simulink model "Configuration3Code"  (R2021a)
settings: Solver=ode23t  StartTime=0.0  StopTime=60.1  FixedStep=0.05  RelTol=1e-3  EnableMultiTasking=on
model workspace (MAT data in the model file):
  mapForSim : object (value not decoded)
  occGrid : robotics.BinaryOccupancyGrid (value not decoded)
undefined symbols (not defined in the file): cellPose, FloorSurface, isoPoses, objectLevel, objectTypeArray, platformPoses, PlowSurface, Ref, RobotSurface, WallSurface, X, Y, Z
libraries: sm_lib x308, nesl_utility x151, simulink x70, RP_Simulator_Components x4
(part 15 of 15)

== matlab function Configuration3Code/BEST Robotics 2021 Game (Double-Click)/Objects/Object11/MATLAB Function ==
  settings: updateMethod=DISCRETE
  data: latch input; scoreLevel input; inuse input; target input; time input; objPoseX output; robotPoseX input; robotPoseY input; objPoseY output; latched output; initPose parameter; objId parameter; objectType output; endType output; objectTypeArray parameter; gameTime parameter; platformPoses parameter; objectLevel parameter
function [objPoseX, objPoseY, latched, objectType,endType] = latchObject(latch,scoreLevel, inuse, target, time, robotPoseX, robotPoseY, initPose, objId, objectTypeArray, gameTime, platformPoses, objectLevel)
persistent stateX stateY level pickup
if isempty(stateX)
    stateX=initPose(1);
    stateY=initPose(2);
    level=objectLevel;
    pickup=0;
end

if ~latch
     pickup=0;
    if level && ((stateX > platformPoses(1,1)-0.21 && stateX < platformPoses(1,1)+0.21...
            && stateY > platformPoses(1,2)-0.21 && stateY < platformPoses(1,2) +0.21) || ...
            (stateX > platformPoses(2,1)-0.21 && stateX < platformPoses(2,1)+0.21...
            && stateY > platformPoses(2,2)-0.21 && stateY < platformPoses(2,2) +0.21))
        latched=0.2;
    else
        level=0;
        latched=0;
    end
elseif pickup
    stateX=robotPoseX;
    stateY=robotPoseY;
    level=scoreLevel;
    latched=0.15 +level*0.2;
elseif ~inuse && latch && target == objId && ...
        sqrt((stateX-robotPoseX)^2+(stateY-robotPoseY)^2) < 0.08 && scoreLevel==level
    
        pickup=1;
        latched=0.15;
else
   if level && ((stateX > platformPoses(1,1)-0.21 && stateX < platformPoses(1,1)+0.21...
            && stateY > platformPoses(1,2)-0.21 && stateY < platformPoses(1,2) +0.21) || ...
            (stateX > platformPoses(2,1)-0.21 && stateX < platformPoses(2,1)+0.21...
            && stateY > platformPoses(2,2)-0.21 && stateY < platformPoses(2,2) +0.21))
        latched=0.2;
    else
        level=0;
        latched=0;
    end
end
if sqrt((stateX-robotPoseX)^2+(stateY-robotPoseY)^2) < 0.1 && scoreLevel==level
    objectType=objectTypeArray(objId);
else
    objectType=nan;
end

if time > gameTime
    endType=objectTypeArray(objId)+1;
else
    endType=0;
end

objPoseX=stateX;
objPoseY=stateY;

== matlab function Configuration3Code/BEST Robotics 2021 Game (Double-Click)/Objects/Object12/MATLAB Function ==
  settings: updateMethod=DISCRETE
  data: latch input; scoreLevel input; inuse input; target input; time input; objPoseX output; robotPoseX input; robotPoseY input; objPoseY output; latched output; initPose parameter; objId parameter; objectType output; endType output; objectTypeArray parameter; gameTime parameter; platformPoses parameter; objectLevel parameter
function [objPoseX, objPoseY, latched, objectType,endType] = latchObject(latch,scoreLevel, inuse, target, time, robotPoseX, robotPoseY, initPose, objId, objectTypeArray, gameTime, platformPoses, objectLevel)
persistent stateX stateY level pickup
if isempty(stateX)
    stateX=initPose(1);
    stateY=initPose(2);
    level=objectLevel;
    pickup=0;
end

if ~latch
     pickup=0;
    if level && ((stateX > platformPoses(1,1)-0.21 && stateX < platformPoses(1,1)+0.21...
            && stateY > platformPoses(1,2)-0.21 && stateY < platformPoses(1,2) +0.21) || ...
            (stateX > platformPoses(2,1)-0.21 && stateX < platformPoses(2,1)+0.21...
            && stateY > platformPoses(2,2)-0.21 && stateY < platformPoses(2,2) +0.21))
        latched=0.2;
    else
        level=0;
        latched=0;
    end
elseif pickup
    stateX=robotPoseX;
    stateY=robotPoseY;
    level=scoreLevel;
    latched=0.15 +level*0.2;
elseif ~inuse && latch && target == objId && ...
        sqrt((stateX-robotPoseX)^2+(stateY-robotPoseY)^2) < 0.08 && scoreLevel==level
    
        pickup=1;
        latched=0.15;
else
   if level && ((stateX > platformPoses(1,1)-0.21 && stateX < platformPoses(1,1)+0.21...
            && stateY > platformPoses(1,2)-0.21 && stateY < platformPoses(1,2) +0.21) || ...
            (stateX > platformPoses(2,1)-0.21 && stateX < platformPoses(2,1)+0.21...
            && stateY > platformPoses(2,2)-0.21 && stateY < platformPoses(2,2) +0.21))
        latched=0.2;
    else
        level=0;
        latched=0;
    end
end
if sqrt((stateX-robotPoseX)^2+(stateY-robotPoseY)^2) < 0.1 && scoreLevel==level
    objectType=objectTypeArray(objId);
else
    objectType=nan;
end

if time > gameTime
    endType=objectTypeArray(objId)+1;
else
    endType=0;
end

objPoseX=stateX;
objPoseY=stateY;

== matlab function Configuration3Code/BEST Robotics 2021 Game (Double-Click)/Objects/Object13/MATLAB Function ==
  settings: updateMethod=DISCRETE
  data: latch input; scoreLevel input; inuse input; target input; time input; objPoseX output; robotPoseX input; robotPoseY input; objPoseY output; latched output; initPose parameter; objId parameter; objectType output; endType output; objectTypeArray parameter; gameTime parameter; platformPoses parameter; objectLevel parameter
function [objPoseX, objPoseY, latched, objectType,endType] = latchObject(latch,scoreLevel, inuse, target, time, robotPoseX, robotPoseY, initPose, objId, objectTypeArray, gameTime, platformPoses, objectLevel)
persistent stateX stateY level pickup
if isempty(stateX)
    stateX=initPose(1);
    stateY=initPose(2);
    level=objectLevel;
    pickup=0;
end

if ~latch
     pickup=0;
    if level && ((stateX > platformPoses(1,1)-0.21 && stateX < platformPoses(1,1)+0.21...
            && stateY > platformPoses(1,2)-0.21 && stateY < platformPoses(1,2) +0.21) || ...
            (stateX > platformPoses(2,1)-0.21 && stateX < platformPoses(2,1)+0.21...
            && stateY > platformPoses(2,2)-0.21 && stateY < platformPoses(2,2) +0.21))
        latched=0.2;
    else
        level=0;
        latched=0;
    end
elseif pickup
    stateX=robotPoseX;
    stateY=robotPoseY;
    level=scoreLevel;
    latched=0.15 +level*0.2;
elseif ~inuse && latch && target == objId && ...
        sqrt((stateX-robotPoseX)^2+(stateY-robotPoseY)^2) < 0.08 && scoreLevel==level
    
        pickup=1;
        latched=0.15;
else
   if level && ((stateX > platformPoses(1,1)-0.21 && stateX < platformPoses(1,1)+0.21...
            && stateY > platformPoses(1,2)-0.21 && stateY < platformPoses(1,2) +0.21) || ...
            (stateX > platformPoses(2,1)-0.21 && stateX < platformPoses(2,1)+0.21...
            && stateY > platformPoses(2,2)-0.21 && stateY < platformPoses(2,2) +0.21))
        latched=0.2;
    else
        level=0;
        latched=0;
    end
end
if sqrt((stateX-robotPoseX)^2+(stateY-robotPoseY)^2) < 0.1 && scoreLevel==level
    objectType=objectTypeArray(objId);
else
    objectType=nan;
end

if time > gameTime
    endType=objectTypeArray(objId)+1;
else
    endType=0;
end

objPoseX=stateX;
objPoseY=stateY;

== matlab function Configuration3Code/BEST Robotics 2021 Game (Double-Click)/Objects/Object14/MATLAB Function ==
  settings: updateMethod=DISCRETE
  data: latch input; scoreLevel input; inuse input; target input; time input; objPoseX output; robotPoseX input; robotPoseY input; objPoseY output; latched output; initPose parameter; objId parameter; objectType output; endType output; objectTypeArray parameter; gameTime parameter; platformPoses parameter; objectLevel parameter
function [objPoseX, objPoseY, latched, objectType,endType] = latchObject(latch,scoreLevel, inuse, target, time, robotPoseX, robotPoseY, initPose, objId, objectTypeArray, gameTime, platformPoses, objectLevel)
persistent stateX stateY level pickup
if isempty(stateX)
    stateX=initPose(1);
    stateY=initPose(2);
    level=objectLevel;
    pickup=0;
end

if ~latch
     pickup=0;
    if level && ((stateX > platformPoses(1,1)-0.21 && stateX < platformPoses(1,1)+0.21...
            && stateY > platformPoses(1,2)-0.21 && stateY < platformPoses(1,2) +0.21) || ...
            (stateX > platformPoses(2,1)-0.21 && stateX < platformPoses(2,1)+0.21...
            && stateY > platformPoses(2,2)-0.21 && stateY < platformPoses(2,2) +0.21))
        latched=0.2;
    else
        level=0;
        latched=0;
    end
elseif pickup
    stateX=robotPoseX;
    stateY=robotPoseY;
    level=scoreLevel;
    latched=0.15 +level*0.2;
elseif ~inuse && latch && target == objId && ...
        sqrt((stateX-robotPoseX)^2+(stateY-robotPoseY)^2) < 0.08 && scoreLevel==level
    
        pickup=1;
        latched=0.15;
else
   if level && ((stateX > platformPoses(1,1)-0.21 && stateX < platformPoses(1,1)+0.21...
            && stateY > platformPoses(1,2)-0.21 && stateY < platformPoses(1,2) +0.21) || ...
            (stateX > platformPoses(2,1)-0.21 && stateX < platformPoses(2,1)+0.21...
            && stateY > platformPoses(2,2)-0.21 && stateY < platformPoses(2,2) +0.21))
        latched=0.2;
    else
        level=0;
        latched=0;
    end
end
if sqrt((stateX-robotPoseX)^2+(stateY-robotPoseY)^2) < 0.1 && scoreLevel==level
    objectType=objectTypeArray(objId);
else
    objectType=nan;
end

if time > gameTime
    endType=objectTypeArray(objId)+1;
else
    endType=0;
end

objPoseX=stateX;
objPoseY=stateY;

== matlab function Configuration3Code/BEST Robotics 2021 Game (Double-Click)/Objects/Object15/MATLAB Function ==
  settings: updateMethod=DISCRETE
  data: latch input; scoreLevel input; inuse input; target input; time input; objPoseX output; robotPoseX input; robotPoseY input; objPoseY output; latched output; initPose parameter; objId parameter; objectType output; endType output; objectTypeArray parameter; gameTime parameter; platformPoses parameter; objectLevel parameter
function [objPoseX, objPoseY, latched, objectType,endType] = latchObject(latch,scoreLevel, inuse, target, time, robotPoseX, robotPoseY, initPose, objId, objectTypeArray, gameTime, platformPoses, objectLevel)
persistent stateX stateY level pickup
if isempty(stateX)
    stateX=initPose(1);
    stateY=initPose(2);
    level=objectLevel;
    pickup=0;
end

if ~latch
     pickup=0;
    if level && ((stateX > platformPoses(1,1)-0.21 && stateX < platformPoses(1,1)+0.21...
            && stateY > platformPoses(1,2)-0.21 && stateY < platformPoses(1,2) +0.21) || ...
            (stateX > platformPoses(2,1)-0.21 && stateX < platformPoses(2,1)+0.21...
            && stateY > platformPoses(2,2)-0.21 && stateY < platformPoses(2,2) +0.21))
        latched=0.2;
    else
        level=0;
        latched=0;
    end
elseif pickup
    stateX=robotPoseX;
    stateY=robotPoseY;
    level=scoreLevel;
    latched=0.15 +level*0.2;
elseif ~inuse && latch && target == objId && ...
        sqrt((stateX-robotPoseX)^2+(stateY-robotPoseY)^2) < 0.08 && scoreLevel==level
    
        pickup=1;
        latched=0.15;
else
   if level && ((stateX > platformPoses(1,1)-0.21 && stateX < platformPoses(1,1)+0.21...
            && stateY > platformPoses(1,2)-0.21 && stateY < platformPoses(1,2) +0.21) || ...
            (stateX > platformPoses(2,1)-0.21 && stateX < platformPoses(2,1)+0.21...
            && stateY > platformPoses(2,2)-0.21 && stateY < platformPoses(2,2) +0.21))
        latched=0.2;
    else
        level=0;
        latched=0;
    end
end
if sqrt((stateX-robotPoseX)^2+(stateY-robotPoseY)^2) < 0.1 && scoreLevel==level
    objectType=objectTypeArray(objId);
else
    objectType=nan;
end

if time > gameTime
    endType=objectTypeArray(objId)+1;
else
    endType=0;
end

objPoseX=stateX;
objPoseY=stateY;

== matlab function Configuration3Code/BEST Robotics 2021 Game (Double-Click)/Objects/Object16/MATLAB Function ==
  settings: updateMethod=DISCRETE
  data: latch input; scoreLevel input; inuse input; target input; time input; objPoseX output; robotPoseX input; robotPoseY input; objPoseY output; latched output; initPose parameter; objId parameter; objectType output; endType output; objectTypeArray parameter; gameTime parameter; platformPoses parameter; objectLevel parameter
function [objPoseX, objPoseY, latched, objectType,endType] = latchObject(latch,scoreLevel, inuse, target, time, robotPoseX, robotPoseY, initPose, objId, objectTypeArray, gameTime, platformPoses, objectLevel)
persistent stateX stateY level pickup
if isempty(stateX)
    stateX=initPose(1);
    stateY=initPose(2);
    level=objectLevel;
    pickup=0;
end

if ~latch
     pickup=0;
    if level && ((stateX > platformPoses(1,1)-0.21 && stateX < platformPoses(1,1)+0.21...
            && stateY > platformPoses(1,2)-0.21 && stateY < platformPoses(1,2) +0.21) || ...
            (stateX > platformPoses(2,1)-0.21 && stateX < platformPoses(2,1)+0.21...
            && stateY > platformPoses(2,2)-0.21 && stateY < platformPoses(2,2) +0.21))
        latched=0.2;
    else
        level=0;
        latched=0;
    end
elseif pickup
    stateX=robotPoseX;
    stateY=robotPoseY;
    level=scoreLevel;
    latched=0.15 +level*0.2;
elseif ~inuse && latch && target == objId && ...
        sqrt((stateX-robotPoseX)^2+(stateY-robotPoseY)^2) < 0.08 && scoreLevel==level
    
        pickup=1;
        latched=0.15;
else
   if level && ((stateX > platformPoses(1,1)-0.21 && stateX < platformPoses(1,1)+0.21...
            && stateY > platformPoses(1,2)-0.21 && stateY < platformPoses(1,2) +0.21) || ...
            (stateX > platformPoses(2,1)-0.21 && stateX < platformPoses(2,1)+0.21...
            && stateY > platformPoses(2,2)-0.21 && stateY < platformPoses(2,2) +0.21))
        latched=0.2;
    else
        level=0;
        latched=0;
    end
end
if sqrt((stateX-robotPoseX)^2+(stateY-robotPoseY)^2) < 0.1 && scoreLevel==level
    objectType=objectTypeArray(objId);
else
    objectType=nan;
end

if time > gameTime
    endType=objectTypeArray(objId)+1;
else
    endType=0;
end

objPoseX=stateX;
objPoseY=stateY;

== matlab function Configuration3Code/BEST Robotics 2021 Game (Double-Click)/Objects/Object17/MATLAB Function ==
  settings: updateMethod=DISCRETE
  data: latch input; scoreLevel input; inuse input; target input; time input; objPoseX output; robotPoseX input; robotPoseY input; objPoseY output; latched output; initPose parameter; objId parameter; objectType output; endType output; objectTypeArray parameter; gameTime parameter; platformPoses parameter; objectLevel parameter
function [objPoseX, objPoseY, latched, objectType,endType] = latchObject(latch,scoreLevel, inuse, target, time, robotPoseX, robotPoseY, initPose, objId, objectTypeArray, gameTime, platformPoses, objectLevel)
persistent stateX stateY level pickup
if isempty(stateX)
    stateX=initPose(1);
    stateY=initPose(2);
    level=objectLevel;
    pickup=0;
end

if ~latch
     pickup=0;
    if level && ((stateX > platformPoses(1,1)-0.21 && stateX < platformPoses(1,1)+0.21...
            && stateY > platformPoses(1,2)-0.21 && stateY < platformPoses(1,2) +0.21) || ...
            (stateX > platformPoses(2,1)-0.21 && stateX < platformPoses(2,1)+0.21...
            && stateY > platformPoses(2,2)-0.21 && stateY < platformPoses(2,2) +0.21))
        latched=0.2;
    else
        level=0;
        latched=0;
    end
elseif pickup
    stateX=robotPoseX;
    stateY=robotPoseY;
    level=scoreLevel;
    latched=0.15 +level*0.2;
elseif ~inuse && latch && target == objId && ...
        sqrt((stateX-robotPoseX)^2+(stateY-robotPoseY)^2) < 0.08 && scoreLevel==level
    
        pickup=1;
        latched=0.15;
else
   if level && ((stateX > platformPoses(1,1)-0.21 && stateX < platformPoses(1,1)+0.21...
            && stateY > platformPoses(1,2)-0.21 && stateY < platformPoses(1,2) +0.21) || ...
            (stateX > platformPoses(2,1)-0.21 && stateX < platformPoses(2,1)+0.21...
            && stateY > platformPoses(2,2)-0.21 && stateY < platformPoses(2,2) +0.21))
        latched=0.2;
    else
        level=0;
        latched=0;
    end
end
if sqrt((stateX-robotPoseX)^2+(stateY-robotPoseY)^2) < 0.1 && scoreLevel==level
    objectType=objectTypeArray(objId);
else
    objectType=nan;
end

if time > gameTime
    endType=objectTypeArray(objId)+1;
else
    endType=0;
end

objPoseX=stateX;
objPoseY=stateY;

== matlab function Configuration3Code/BEST Robotics 2021 Game (Double-Click)/Objects/Object18/MATLAB Function ==
  settings: updateMethod=DISCRETE
  data: latch input; scoreLevel input; inuse input; target input; time input; objPoseX output; robotPoseX input; robotPoseY input; objPoseY output; latched output; initPose parameter; objId parameter; objectType output; endType output; objectTypeArray parameter; gameTime parameter; platformPoses parameter; objectLevel parameter
function [objPoseX, objPoseY, latched, objectType,endType] = latchObject(latch,scoreLevel, inuse, target, time, robotPoseX, robotPoseY, initPose, objId, objectTypeArray, gameTime, platformPoses, objectLevel)
persistent stateX stateY level pickup
if isempty(stateX)
    stateX=initPose(1);
    stateY=initPose(2);
    level=objectLevel;
    pickup=0;
end

if ~latch
     pickup=0;
    if level && ((stateX > platformPoses(1,1)-0.21 && stateX < platformPoses(1,1)+0.21...
            && stateY > platformPoses(1,2)-0.21 && stateY < platformPoses(1,2) +0.21) || ...
            (stateX > platformPoses(2,1)-0.21 && stateX < platformPoses(2,1)+0.21...
            && stateY > platformPoses(2,2)-0.21 && stateY < platformPoses(2,2) +0.21))
        latched=0.2;
    else
        level=0;
        latched=0;
    end
elseif pickup
    stateX=robotPoseX;
    stateY=robotPoseY;
    level=scoreLevel;
    latched=0.15 +level*0.2;
elseif ~inuse && latch && target == objId && ...
        sqrt((stateX-robotPoseX)^2+(stateY-robotPoseY)^2) < 0.08 && scoreLevel==level
    
        pickup=1;
        latched=0.15;
else
   if level && ((stateX > platformPoses(1,1)-0.21 && stateX < platformPoses(1,1)+0.21...
            && stateY > platformPoses(1,2)-0.21 && stateY < platformPoses(1,2) +0.21) || ...
            (stateX > platformPoses(2,1)-0.21 && stateX < platformPoses(2,1)+0.21...
            && stateY > platformPoses(2,2)-0.21 && stateY < platformPoses(2,2) +0.21))
        latched=0.2;
    else
        level=0;
        latched=0;
    end
end
if sqrt((stateX-robotPoseX)^2+(stateY-robotPoseY)^2) < 0.1 && scoreLevel==level
    objectType=objectTypeArray(objId);
else
    objectType=nan;
end

if time > gameTime
    endType=objectTypeArray(objId)+1;
else
    endType=0;
end

objPoseX=stateX;
objPoseY=stateY;

== matlab function Configuration3Code/BEST Robotics 2021 Game (Double-Click)/Objects/Object19/MATLAB Function ==
  settings: updateMethod=DISCRETE
  data: latch input; scoreLevel input; inuse input; target input; time input; objPoseX output; robotPoseX input; robotPoseY input; objPoseY output; latched output; initPose parameter; objId parameter; objectType output; endType output; objectTypeArray parameter; gameTime parameter; platformPoses parameter; objectLevel parameter
function [objPoseX, objPoseY, latched, objectType,endType] = latchObject(latch,scoreLevel, inuse, target, time, robotPoseX, robotPoseY, initPose, objId, objectTypeArray, gameTime, platformPoses, objectLevel)
persistent stateX stateY level pickup
if isempty(stateX)
    stateX=initPose(1);
    stateY=initPose(2);
    level=objectLevel;
    pickup=0;
end

if ~latch
     pickup=0;
    if level && ((stateX > platformPoses(1,1)-0.21 && stateX < platformPoses(1,1)+0.21...
            && stateY > platformPoses(1,2)-0.21 && stateY < platformPoses(1,2) +0.21) || ...
            (stateX > platformPoses(2,1)-0.21 && stateX < platformPoses(2,1)+0.21...
            && stateY > platformPoses(2,2)-0.21 && stateY < platformPoses(2,2) +0.21))
        latched=0.2;
    else
        level=0;
        latched=0;
    end
elseif pickup
    stateX=robotPoseX;
    stateY=robotPoseY;
    level=scoreLevel;
    latched=0.15 +level*0.2;
elseif ~inuse && latch && target == objId && ...
        sqrt((stateX-robotPoseX)^2+(stateY-robotPoseY)^2) < 0.08 && scoreLevel==level
    
        pickup=1;
        latched=0.15;
else
   if level && ((stateX > platformPoses(1,1)-0.21 && stateX < platformPoses(1,1)+0.21...
            && stateY > platformPoses(1,2)-0.21 && stateY < platformPoses(1,2) +0.21) || ...
            (stateX > platformPoses(2,1)-0.21 && stateX < platformPoses(2,1)+0.21...
            && stateY > platformPoses(2,2)-0.21 && stateY < platformPoses(2,2) +0.21))
        latched=0.2;
    else
        level=0;
        latched=0;
    end
end
if sqrt((stateX-robotPoseX)^2+(stateY-robotPoseY)^2) < 0.1 && scoreLevel==level
    objectType=objectTypeArray(objId);
else
    objectType=nan;
end

if time > gameTime
    endType=objectTypeArray(objId)+1;
else
    endType=0;
end

objPoseX=stateX;
objPoseY=stateY;

== matlab function Configuration3Code/BEST Robotics 2021 Game (Double-Click)/Objects/Object20/MATLAB Function ==
  settings: updateMethod=DISCRETE
  data: latch input; scoreLevel input; inuse input; target input; time input; objPoseX output; robotPoseX input; robotPoseY input; objPoseY output; latched output; initPose parameter; objId parameter; objectType output; endType output; objectTypeArray parameter; gameTime parameter; platformPoses parameter; objectLevel parameter
function [objPoseX, objPoseY, latched, objectType,endType] = latchObject(latch,scoreLevel, inuse, target, time, robotPoseX, robotPoseY, initPose, objId, objectTypeArray, gameTime, platformPoses, objectLevel)
persistent stateX stateY level pickup
if isempty(stateX)
    stateX=initPose(1);
    stateY=initPose(2);
    level=objectLevel;
    pickup=0;
end

if ~latch
     pickup=0;
    if level && ((stateX > platformPoses(1,1)-0.21 && stateX < platformPoses(1,1)+0.21...
            && stateY > platformPoses(1,2)-0.21 && stateY < platformPoses(1,2) +0.21) || ...
            (stateX > platformPoses(2,1)-0.21 && stateX < platformPoses(2,1)+0.21...
            && stateY > platformPoses(2,2)-0.21 && stateY < platformPoses(2,2) +0.21))
        latched=0.2;
    else
        level=0;
        latched=0;
    end
elseif pickup
    stateX=robotPoseX;
    stateY=robotPoseY;
    level=scoreLevel;
    latched=0.15 +level*0.2;
elseif ~inuse && latch && target == objId && ...
        sqrt((stateX-robotPoseX)^2+(stateY-robotPoseY)^2) < 0.08 && scoreLevel==level
    
        pickup=1;
        latched=0.15;
else
   if level && ((stateX > platformPoses(1,1)-0.21 && stateX < platformPoses(1,1)+0.21...
            && stateY > platformPoses(1,2)-0.21 && stateY < platformPoses(1,2) +0.21) || ...
            (stateX > platformPoses(2,1)-0.21 && stateX < platformPoses(2,1)+0.21...
            && stateY > platformPoses(2,2)-0.21 && stateY < platformPoses(2,2) +0.21))
        latched=0.2;
    else
        level=0;
        latched=0;
    end
end
if sqrt((stateX-robotPoseX)^2+(stateY-robotPoseY)^2) < 0.1 && scoreLevel==level
    objectType=objectTypeArray(objId);
else
    objectType=nan;
end

if time > gameTime
    endType=objectTypeArray(objId)+1;
else
    endType=0;
end

objPoseX=stateX;
objPoseY=stateY;

== matlab function Configuration3Code/BEST Robotics 2021 Game (Double-Click)/Game Control/ScoringBlock ==
  data: GameResults input; FinalScore output; BlueFence output; RedFence output; GreenFence output; YellowFence output; Pole1 output; Pole2 output; Pole3 output; TrashPile output; ReuseBin output; RecycleBin output
function [FinalScore, BlueFence, RedFence, GreenFence, YellowFence, Pole1, Pole2, Pole3, TrashPile, ReuseBin, RecycleBin]  = ScoreObjects(GameResults)

ScoreLoc = [
    48.6220   48.6220  62.4015  62.4015;...  %Blue 1
    48.6220   34.8425  62.4015  48.6220;...  %Red 2
    48.6220   21.0630  62.4015  34.8425;...  %Green 3
    48.6220    7.2835  62.4015  21.0630;...  %Yellow 4
    -8.4646   49.2125   7.6772  58.6613;...  %Recycle 5
    45.8661  -58.6613  62.0078 -49.2125;...  %Reuse 6
    -82.6770 -9.8425  -62.9920   9.8425;...  %TrashPile 7
    16.7323   15.9449  22.6378  21.8504;...  %LightBase1 8
    -26.5748 -54.9212 -20.6693 -49.0157;...  %LightBase2 9
    -58.8582  51.7716 -52.9527  57.6771];    %LightBase3 10

%     1.235	1.235	1.585	1.585;...   %Blue 1
%     1.235	0.885	1.585	1.235;...   %Red 2
%     1.235	0.535	1.585	0.885;...   %Green 3
%     1.235	0.185	1.585	0.535;...   %Yellow 4
%     -0.215	1.250	0.195	1.575;...   %Recycle 5
%     1.165	-1.575	1.575	-1.250;...  %Reuse 6
%     -2.1	-0.25	-1.6	0.25;...    %TrashPile 7
%     0.425	0.405	0.575	0.555;...   %LightBase1 8
%     -0.675	-1.395	-0.525	-1.245;...  %LightBase2 9
%     -1.495	1.315	-1.345	1.465];     %LightBase3 10

BlueFence = 0;
RedFence = 0;
GreenFence = 0;
YellowFence = 0;
Pole1 = 0;
Pole2 = 0;
Pole3 = 0;
TrashPile = 0;
ReuseBin = 0;
RecycleBin = 0;

BlueFence   = 20 * ( all(GameResults(1,1:2) >= ScoreLoc(1,1:2) & GameResults(1,1:2) <= ScoreLoc(1,3:4)) );
RedFence    = 20 * ( all(GameResults(2,1:2) >= ScoreLoc(2,1:2) & GameResults(2,1:2) <= ScoreLoc(2,3:4)) );
GreenFence  = 20 * ( all(GameResults(3,1:2) >= ScoreLoc(3,1:2) & GameResults(3,1:2) <= ScoreLoc(3,3:4)) );
YellowFence = 20 * ( all(GameResults(4,1:2) >= ScoreLoc(4,1:2) & GameResults(4,1:2) <= ScoreLoc(4,3:4)) );

Pole1     = 15 * ( all(GameResults(22,1:2) >= ScoreLoc(8,1:2)  & GameResults(22,1:2) <= ScoreLoc(8,3:4) ) || ...
                   all(GameResults(22,1:2) >= ScoreLoc(9,1:2)  & GameResults(22,1:2) <= ScoreLoc(9,3:4) ) || ...
                   all(GameResults(22,1:2) >= ScoreLoc(10,1:2) & GameResults(22,1:2) <= ScoreLoc(10,3:4))    ...
                 );  %add & (ObjType=NAN) ?
                 
Pole2     = 15 * ( all(GameResults(23,1:2) >= ScoreLoc(8,1:2)  & GameResults(23,1:2) <= ScoreLoc(8,3:4) ) || ...
                   all(GameResults(23,1:2) >= ScoreLoc(9,1:2)  & GameResults(23,1:2) <= ScoreLoc(9,3:4) ) || ...
                   all(GameResults(23,1:2) >= ScoreLoc(10,1:2) & GameResults(23,1:2) <= ScoreLoc(10,3:4))    ...
                 );
                 
Pole3     = 15 * ( all(GameResults(24,1:2) >= ScoreLoc(8,1:2)  & GameResults(24,1:2) <= ScoreLoc(8,3:4) ) || ...
                   all(GameResults(24,1:2) >= ScoreLoc(9,1:2)  & GameResults(24,1:2) <= ScoreLoc(9,3:4) ) || ...
                   all(GameResults(24,1:2) >= ScoreLoc(10,1:2) & GameResults(24,1:2) <= ScoreLoc(10,3:4))    ...
                 );

for i=5:20
    switch GameResults(i,4)
        case 1   % trash
          TrashPile = TrashPile   + 10 * ( all(GameResults(i,1:2) >= ScoreLoc(7,1:2) & GameResults(i,1:2) <= ScoreLoc(7,3:4)) ); 
        case 2   % Reuse  (must have level=1)
          ReuseBin = ReuseBin     + 20 * (GameResults(i,3)==0.5) * ( all(GameResults(i,1:2) >= ScoreLoc(6,1:2) & GameResults(i,1:2) <= ScoreLoc(6,3:4)) ); 
        case 3   % trash
          TrashPile = TrashPile   + 10 * ( all(GameResults(i,1:2) >= ScoreLoc(7,1:2) & GameResults(i,1:2) <= ScoreLoc(7,3:4)) ); 
        case 4   % Recycle
          RecycleBin = RecycleBin + 25 * (GameResults(i,3)==0.5) * ( all(GameResults(i,1:2) >= ScoreLoc(5,1:2) & GameResults(i,1:2) <= ScoreLoc(5,3:4)) ); 
        case 5   % Reuse
          ReuseBin = ReuseBin     + 20 * (GameResults(i,3)==0.5) * ( all(GameResults(i,1:2) >= ScoreLoc(6,1:2) & GameResults(i,1:2) <= ScoreLoc(6,3:4)) ); 
        case 6   % Recycle
          RecycleBin = RecycleBin + 25 * (GameResults(i,3)==0.5) * ( all(GameResults(i,1:2) >= ScoreLoc(5,1:2) & GameResults(i,1:2) <= ScoreLoc(5,3:4)) ); 
        case 7   % Reuse
          ReuseBin = ReuseBin     + 20 * (GameResults(i,3)==0.5) * ( all(GameResults(i,1:2) >= ScoreLoc(6,1:2) & GameResults(i,1:2) <= ScoreLoc(6,3:4)) ); 
        case 8   % Recycle
          RecycleBin = RecycleBin + 25 * (GameResults(i,3)==0.5) * ( all(GameResults(i,1:2) >= ScoreLoc(5,1:2) & GameResults(i,1:2) <= ScoreLoc(5,3:4)) ); 
        otherwise
    end 
    
FinalScore = BlueFence + RedFence + GreenFence + YellowFence + Pole1 + Pole2 + Pole3 + TrashPile + ReuseBin + RecycleBin;

end

== matlab function Configuration3Code/BEST Robotics 2021 Game (Double-Click)/Objects/MATLAB Function2 ==
  data: robotPose input; cellPoses input; cellTarget output
function cellTarget = findTarget(robotPose, cellPoses)


eucDist=sqrt((cellPoses(:,1)-robotPose(1)).^2+(cellPoses(:,2)-robotPose(2)).^2);
[~,cellIdx]=min(eucDist);
cellTarget = cellIdx;

== matlab function Configuration3Code/BEST Robotics 2021 Game (Double-Click)/Light poles/Light pole/MATLAB Function ==
  settings: updateMethod=DISCRETE
  data: drop input; level input; objPoseX output; robotPoseX input; robotPoseY input; objPoseY output; lightpole output
function [objPoseX, objPoseY, lightpole] = latchObject(drop, level, robotPoseX, robotPoseY)
persistent stateX stateY stateZ prevDrop dropped
if isempty(stateX)
    stateX=robotPoseX+0.14;
    stateY=robotPoseY;
    stateZ=0.15;
    prevDrop=0;
    dropped=0;
end

if drop && prevDrop && ~dropped
    stateX=robotPoseX;
    stateY=robotPoseY;
    stateZ=level*0.4;
    objPoseX=robotPoseX;
    objPoseY=robotPoseY;
    dropped=1;
elseif dropped
    objPoseX=stateX;
    objPoseY=stateY;

else
    objPoseX=robotPoseX+0.14;
    objPoseY=robotPoseY;
end
prevDrop=drop;
lightpole=stateZ;

== matlab function Configuration3Code/BEST Robotics 2021 Game (Double-Click)/Light poles/Light pole2/MATLAB Function1 ==
  settings: updateMethod=DISCRETE
  data: drop input; level input; objPoseX output; robotPoseX input; robotPoseY input; objPoseY output; lightpole output
function [objPoseX, objPoseY, lightpole] = latchObject(drop, level, robotPoseX, robotPoseY)
persistent stateX stateY stateZ prevDrop dropped
if isempty(stateX)
    stateX=robotPoseX+0.14;
    stateY=robotPoseY;
    stateZ=0.15;
    prevDrop=0;
    dropped=0;
end

if drop && prevDrop && ~dropped
    stateX=robotPoseX;
    stateY=robotPoseY;
    stateZ=level*0.4;
    objPoseX=robotPoseX;
    objPoseY=robotPoseY;
    dropped=1;
elseif dropped
    objPoseX=stateX;
    objPoseY=stateY;

else
    objPoseX=robotPoseX-0.11;
    objPoseY=robotPoseY+0.11;
end
prevDrop=drop;
lightpole=stateZ;

== matlab function Configuration3Code/BEST Robotics 2021 Game (Double-Click)/Light poles/Light pole1/MATLAB Function1 ==
  settings: updateMethod=DISCRETE
  data: drop input; level input; objPoseX output; robotPoseX input; robotPoseY input; objPoseY output; lightpole output
function [objPoseX, objPoseY, lightpole] = latchObject(drop, level, robotPoseX, robotPoseY)
persistent stateX stateY stateZ prevDrop dropped
if isempty(stateX)
    stateX=robotPoseX+0.14;
    stateY=robotPoseY;
    stateZ=0.15;
    prevDrop=0;
    dropped=0;
end

if drop && prevDrop && ~dropped
    stateX=robotPoseX;
    stateY=robotPoseY;
    stateZ=level*0.4;
    objPoseX=robotPoseX;
    objPoseY=robotPoseY;
    dropped=1;
elseif dropped
    objPoseX=stateX;
    objPoseY=stateY;

else
    objPoseX=robotPoseX-0.11;
    objPoseY=robotPoseY-0.11;
end
prevDrop=drop;
lightpole=stateZ;
